simulink model "frequency_modulation"  (R2020a)
settings: Solver=VariableStepAuto  StartTime=0.0  StopTime=20  RelTol=1e-3
libraries: simulink x7, dspsrcs4 x1
settings Model: Creator=jeeva  LastModifiedBy=jeeva

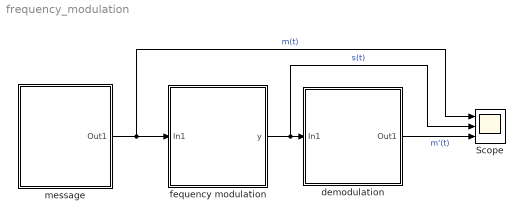
== system frequency_modulation ==
  Scope : Scope  NumInputPorts=3
  demodulation : Subsystem
  fequency modulation : Subsystem
  message : Subsystem
  wires:
  message/1(Out1) -> Scope/1, fequency modulation/1(In1)  "m(t)"
  fequency modulation/1(y) -> Scope/2, demodulation/1(In1)  "s(t)"
  demodulation/1(Out1) -> Scope/3  "m'(t)"

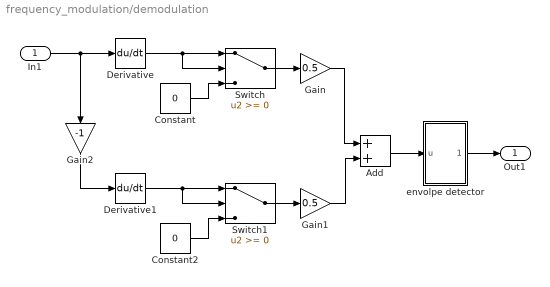
== system frequency_modulation/demodulation ==
  In1 : Inport
  Add : Sum
  Constant : Constant  Value=0
  Constant2 : Constant  Value=0
  Derivative : Derivative
  Derivative1 : Derivative
  Gain : Gain  Gain=0.5
  Gain1 : Gain  Gain=0.5
  Gain2 : Gain  Gain=-1
  Switch : Switch
  Switch1 : Switch
  envolpe detector : Subsystem
  Out1 : Outport
  wires:
  Derivative/1 -> Switch/2, Switch/1
  Gain2/1 -> Derivative1/1
  Switch/1 -> Gain/1
  In1/1 -> Gain2/1, Derivative/1
  envolpe detector/1(Out1) -> Out1/1
  Constant2/1 -> Switch1/3
  Gain/1 -> Add/1
  Constant/1 -> Switch/3
  Derivative1/1 -> Switch1/1, Switch1/2
  Switch1/1 -> Gain1/1
  Gain1/1 -> Add/2
  Add/1 -> envolpe detector/1(u)

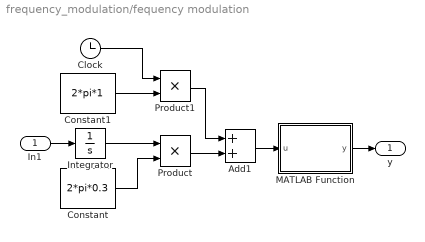
== system frequency_modulation/fequency modulation ==
  In1 : Inport
  Add1 : Sum
  Clock : Clock
  Constant : Constant  Value=2*pi*0.3
  Constant1 : Constant  Value=2*pi*1
  Integrator : Integrator
  MATLAB Function : MATLAB Function  TreatAsAtomicUnit=on
  Product : Product
  Product1 : Product
  y : Outport
  wires:
  Clock/1 -> Product1/1
  Constant1/1 -> Product1/2
  Integrator/1 -> Product/1
  Product1/1 -> Add1/1
  Product/1 -> Add1/2
  Add1/1 -> MATLAB Function/1(u)
  MATLAB Function/1(y) -> y/1
  In1/1 -> Integrator/1
  Constant/1 -> Product/2

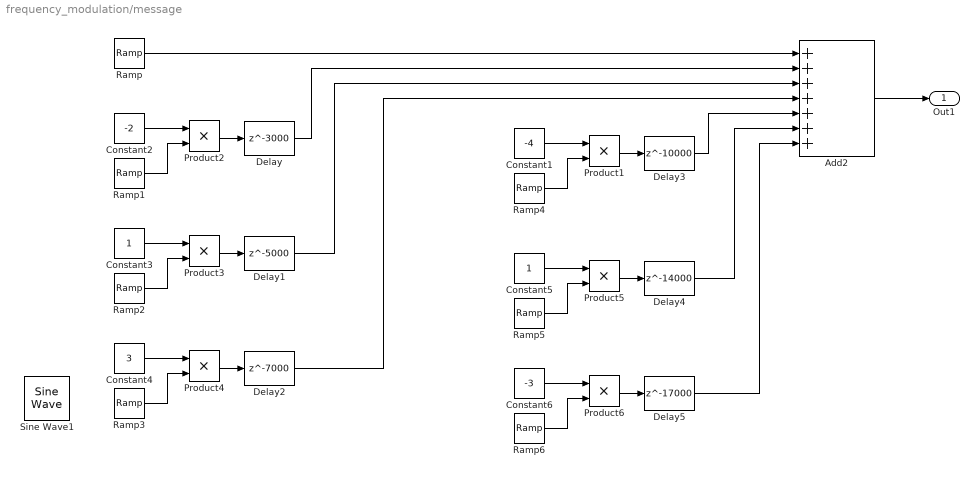
== system frequency_modulation/message ==
  Add2 : Sum  Inputs=+++++++
  Constant1 : Constant  Value=-4
  Constant2 : Constant  Value=-2
  Constant3 : Constant
  Constant4 : Constant  Value=3
  Constant5 : Constant
  Constant6 : Constant  Value=-3
  Delay : Delay  DelayLength=3000
  Delay1 : Delay  DelayLength=5000
  Delay2 : Delay  DelayLength=7000
  Delay3 : Delay  DelayLength=10000
  Delay4 : Delay  DelayLength=14000
  Delay5 : Delay  DelayLength=17000
  Product{1..6} (6 alike) : Product
  Ramp{,1..6} (7 alike) : simulink/Sources/Ramp  slope=5  start=0  InitialOutput=0
  Sine Wave1 : dspsrcs4/Sine Wave  Amplitude=5  Frequency=0.8  Phase=pi/2  SampleMode=Discrete  OutComplex=Real  CompMethod=Trigonometric fcn  TableSize=Speed  SampleTime=1/1000  SamplesPerFrame=1  ResetState=Restart at time zero  OutputFrames=off  dataType=double  wordLen=16  udDataType=sfix(16)  fracBitsMode=Best precision  numFracBits=15  OutDataTypeStr=double  LastOutDataTypeStr=double
  Out1 : Outport
  wires:
  Ramp/1 -> Add2/1
  Product3/1 -> Delay1/1
  Ramp1/1 -> Product2/2
  Constant4/1 -> Product4/1
  Product4/1 -> Delay2/1
  Delay1/1 -> Add2/3
  Ramp3/1 -> Product4/2
  Delay2/1 -> Add2/4
  Product2/1 -> Delay/1
  Constant2/1 -> Product2/1
  Constant3/1 -> Product3/1
  Delay/1 -> Add2/2
  Ramp2/1 -> Product3/2
  Add2/1 -> Out1/1
  Ramp4/1 -> Product1/2
  Product1/1 -> Delay3/1
  Constant1/1 -> Product1/1
  Delay3/1 -> Add2/5
  Constant5/1 -> Product5/1
  Product5/1 -> Delay4/1
  Ramp5/1 -> Product5/2
  Ramp6/1 -> Product6/2
  Product6/1 -> Delay5/1
  Constant6/1 -> Product6/1
  Delay4/1 -> Add2/6
  Delay5/1 -> Add2/7

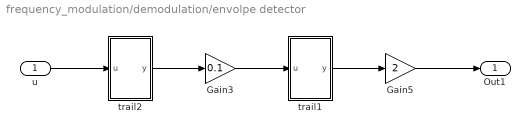
== system frequency_modulation/demodulation/envolpe detector ==
  u : Inport
  Gain3 : Gain  Gain=0.1
  Gain5 : Gain  Gain=2
  trail1 : Subsystem
  trail2 : Subsystem
  Out1 : Outport
  wires:
  Gain3/1 -> trail1/1(u)
  trail1/1(y) -> Gain5/1
  trail2/1(y) -> Gain3/1
  u/1 -> trail2/1(u)
  Gain5/1 -> Out1/1

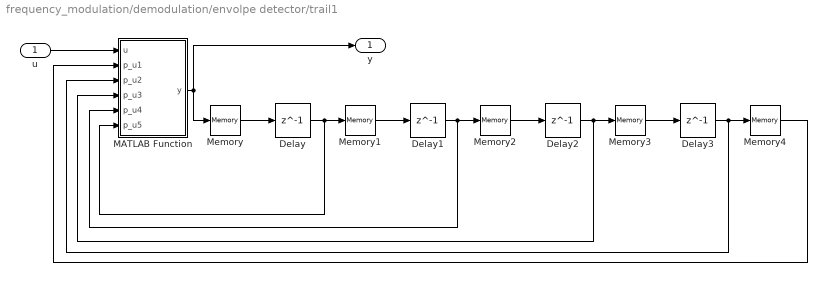
== system frequency_modulation/demodulation/envolpe detector/trail1 ==
  u : Inport
  Delay{,1..3} (4 alike) : Delay  DelayLength=1
  MATLAB Function : MATLAB Function  TreatAsAtomicUnit=on
  Memory{,1..4} (5 alike) : Memory  InheritSampleTime=on
  y : Outport
  wires:
  Delay3/1 -> MATLAB Function/3(p_u2), Memory4/1
  Delay2/1 -> MATLAB Function/4(p_u3), Memory3/1
  Delay/1 -> MATLAB Function/6(p_u5), Memory1/1
  MATLAB Function/1(y) -> y/1, Memory/1
  Memory2/1 -> Delay2/1
  Memory4/1 -> MATLAB Function/2(p_u1)
  Delay1/1 -> MATLAB Function/5(p_u4), Memory2/1
  Memory3/1 -> Delay3/1
  Memory/1 -> Delay/1
  Memory1/1 -> Delay1/1
  u/1 -> MATLAB Function/1(u)

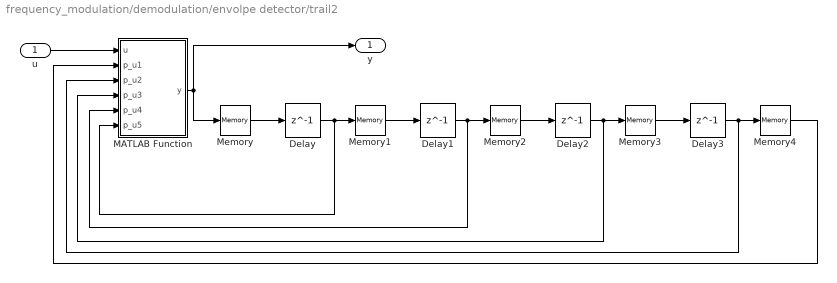
== system frequency_modulation/demodulation/envolpe detector/trail2 ==
  u : Inport
  Delay{,1..3} (4 alike) : Delay  DelayLength=1
  MATLAB Function : MATLAB Function  TreatAsAtomicUnit=on
  Memory{,1..4} (5 alike) : Memory  InheritSampleTime=on
  y : Outport
  wires:
  u/1 -> MATLAB Function/1(u)
  Memory1/1 -> Delay1/1
  Memory/1 -> Delay/1
  Memory3/1 -> Delay3/1
  Delay1/1 -> Memory2/1, MATLAB Function/5(p_u4)
  Memory4/1 -> MATLAB Function/2(p_u1)
  Memory2/1 -> Delay2/1
  MATLAB Function/1(y) -> Memory/1, y/1
  Delay/1 -> Memory1/1, MATLAB Function/6(p_u5)
  Delay2/1 -> Memory3/1, MATLAB Function/4(p_u3)
  Delay3/1 -> Memory4/1, MATLAB Function/3(p_u2)

== matlab function frequency_modulation/demodulation/envolpe detector/trail1/MATLAB Function ==
  data: u input; y output; p_u1 input; p_u2 input; p_u3 input; p_u4 input; p_u5 input
function y = fcn(u, p_u1, p_u2, p_u3, p_u4, p_u5)
%y = 0.5 * u + 0.3 * p_u1 + 0.1 * p_u2 + 0.05 * p_u3 + 0.3 * p_u4 + 0.1 * p_u5;
y = 0.4 * u + 0.3 * p_u1 + 0.2 * p_u2 + 0.05 * p_u3 + 0.3 * p_u4 + 0.1 * p_u5;

== matlab function frequency_modulation/fequency modulation/MATLAB Function ==
  data: u input; y output
function y = fcn(u)

y = cos(u);

== matlab function frequency_modulation/demodulation/envolpe detector/trail2/MATLAB Function ==
  data: u input; y output; p_u1 input; p_u2 input; p_u3 input; p_u4 input; p_u5 input
function y = fcn(u, p_u1, p_u2, p_u3, p_u4, p_u5)

y = 0.9 * u + 0.09 * p_u1 + 0.004 * p_u2 + 0.003 * p_u3 + 0.002 * p_u4 + 0.002 * p_u5;
